simulink model "counter"  (R2021a)
settings: Solver=FixedStepAuto  StartTime=0.0  StopTime=100  FixedStep=1  RelTol=1e-3
settings Model: Creator=Osman  LastModifiedBy=Osman

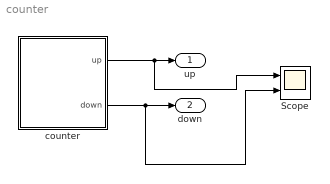
== system counter ==
  Scope : Scope  NumInputPorts=2
  counter : Stateflow chart  TreatAsAtomicUnit=on
  up : Outport
  down : Outport  Port=2
  wires:
  counter/1(up) -> Scope/1, up/1
  counter/2(down) -> Scope/2, down/1

== stateflow chart counter/counter ==
  state reset1
    entry:
    up = 0;
    down = 10;
  state counter
    entry:
    up = up + 1;
    down = down -1;
  (default) -> reset1
  counter -> reset1 [order 1] : [up == 10]
  reset1 -> counter
  counter -> counter [order 2] : after(1,tick)
  data: up output uint16; down output uint16
